simulink model "s20260512_1_quadraped_standup_walk_simulink"  (R2025a)
settings: Solver=FixedStepAuto  StartTime=0.0  StopTime=20  FixedStep=0.001  MaxStep=0.01  RelTol=1e-3
StartFcn:
  | clear functions
values from neighbouring files (symbols this model uses):
  N = size(qr,2)    [animateQuadruped.m]    (also in animateQuadrupedFast.m; animateQuadrupedFastToVideo.m; animateQuadrupedToVideo.m)
  s = norm(axis)    [drawContinuumRobotInstance.m]
  X = 0    [IK_onlyXY.m]    (also in drawContinuumRobotInstance.m = reshape(pts(1,:), size(XC)) + p0(1))
  Y = 0    [IK_onlyXY.m]    (also in drawContinuumRobotInstance.m = reshape(pts(2,:), size(YC)) + p0(2))
  Z = reshape(pts(3,:), size(ZC)) + p0(3)    [drawContinuumRobotInstance.m]
undefined symbols (not defined in the file or in its folder): body_config, leg1_config, leg2_config, leg3_config, leg4_config
libraries: sm_lib x28, nesl_utility x11, simulink x10, snake_single_module_library x5
settings Model: Creator=dperera  LastModifiedBy=dperera
settings SolverCC: ShapePreserveControl=EnableAll  EnableFixedStepZeroCrossing=on
settings OptimizationCC: SimCompilerOptimization=on
settings SFSimCC: UsePrecompiledLibraries=Avoid  SimHardwareAcceleration=native  SimTargetLang=C++  GPUAcceleration=on  SimDLTargetLibrary=cudnn
settings RTWCC: GPUComputeCapability=3.5

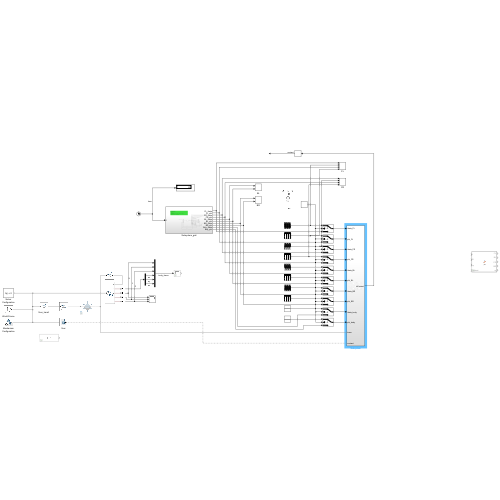
[thumbnail: Simulink's stored preview of the top-level diagram]
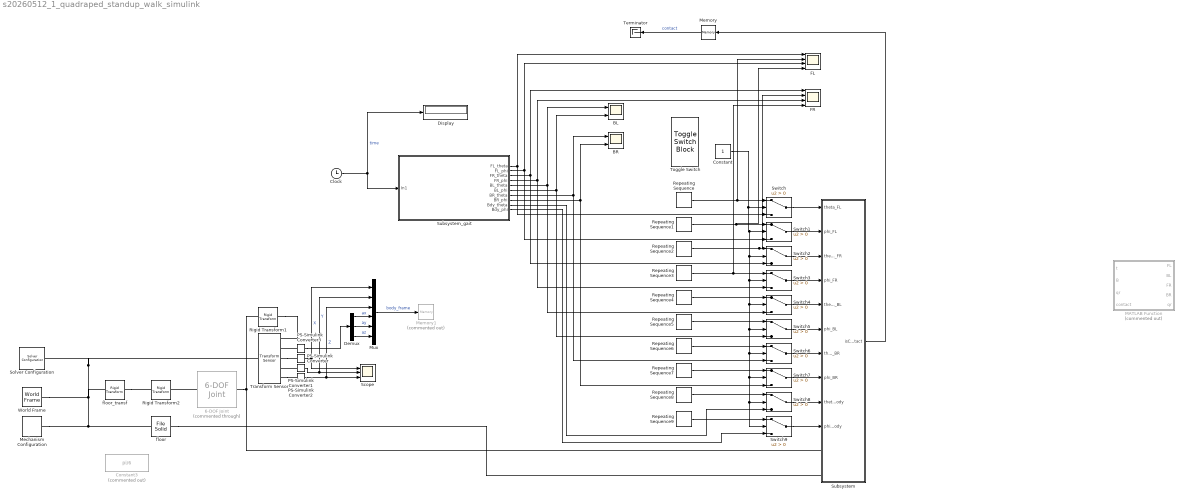
== system s20260512_1_quadraped_standup_walk_simulink ==
  6-DOF Joint : sm_lib/Joints/6-DOF Joint  Commented=through  JointMode=Normal  CompositeWrenchDir=FollowerOnBase  CompositeWrenchFrame=BaseFrame  SenseConstraintForce=off  SenseConstraintTorque=off  SenseTotalForce=off  SenseTotalTorque=off  PxPositionTargetSpecify=off  PxPositionTargetPriority=High  PxPositionTargetValue=0  PxPositionTargetValueUnits=m  PxVelocityTargetSpecify=off  PxVelocityTargetPriority=High  PxVelocityTargetValue=0  PxVelocityTargetValueUnits=m/s  PxEquilibriumPosition=0  PxEquilibriumPositionUnits=m  PxSpringStiffness=0  PxSpringStiffnessUnits=N/m  PxDampingCoefficient=0  PxDampingCoefficientUnits=N/(m/s)  PxLowerLimitSpecify=off  PxLowerLimitBound=-1  PxLowerLimitBoundUnits=m  PxLowerLimitStiffness=1e6  PxLowerLimitStiffnessUnits=N/m  PxLowerLimitDamping=1e3  PxLowerLimitDampingUnits=N/(m/s)  PxLowerLimitTransitionRegionWidth=1e-4  PxLowerLimitTransitionRegionWidthUnits=m  PxUpperLimitSpecify=off  PxUpperLimitBound=1  PxUpperLimitBoundUnits=m  PxUpperLimitStiffness=1e6  PxUpperLimitStiffnessUnits=N/m  PxUpperLimitDamping=1e3  PxUpperLimitDampingUnits=N/(m/s)  PxUpperLimitTransitionRegionWidth=1e-4  PxUpperLimitTransitionRegionWidthUnits=m  PxTorqueActuationMode=NoTorque  PxMotionActuationMode=ComputedMotion  PxSensePosition=off  PxSenseVelocity=off  PxSenseAcceleration=off  PxSenseTorqueForce=off  PxSenseLowerLimitTorqueForce=off  PxSenseUpperLimitTorqueForce=off  PyPositionTargetSpecify=off  PyPositionTargetPriority=High  PyPositionTargetValue=0  PyPositionTargetValueUnits=m  PyVelocityTargetSpecify=off  PyVelocityTargetPriority=High  PyVelocityTargetValue=0  PyVelocityTargetValueUnits=m/s  PyEquilibriumPosition=0  PyEquilibriumPositionUnits=m  PySpringStiffness=0  PySpringStiffnessUnits=N/m  PyDampingCoefficient=0  PyDampingCoefficientUnits=N/(m/s)  PyLowerLimitSpecify=off  PyLowerLimitBound=-1  PyLowerLimitBoundUnits=m  PyLowerLimitStiffness=1e6  PyLowerLimitStiffnessUnits=N/m  PyLowerLimitDamping=1e3  PyLowerLimitDampingUnits=N/(m/s)  PyLowerLimitTransitionRegionWidth=1e-4  PyLowerLimitTransitionRegionWidthUnits=m  PyUpperLimitSpecify=off  PyUpperLimitBound=1  PyUpperLimitBoundUnits=m  PyUpperLimitStiffness=1e6  PyUpperLimitStiffnessUnits=N/m  PyUpperLimitDamping=1e3  PyUpperLimitDampingUnits=N/(m/s)  PyUpperLimitTransitionRegionWidth=1e-4  PyUpperLimitTransitionRegionWidthUnits=m  PyTorqueActuationMode=NoTorque  PyMotionActuationMode=ComputedMotion  PySensePosition=off  PySenseVelocity=off  PySenseAcceleration=off  PySenseTorqueForce=off  PySenseLowerLimitTorqueForce=off  PySenseUpperLimitTorqueForce=off  PzPositionTargetSpecify=off  PzPositionTargetPriority=High  PzPositionTargetValue=0  PzPositionTargetValueUnits=m  PzVelocityTargetSpecify=off  PzVelocityTargetPriority=High  PzVelocityTargetValue=0  PzVelocityTargetValueUnits=m/s  PzEquilibriumPosition=0  PzEquilibriumPositionUnits=m  PzSpringStiffness=0  PzSpringStiffnessUnits=N/m  PzDampingCoefficient=0  PzDampingCoefficientUnits=N/(m/s)  PzLowerLimitSpecify=off  PzLowerLimitBound=-1  PzLowerLimitBoundUnits=m  PzLowerLimitStiffness=1e6  PzLowerLimitStiffnessUnits=N/m  PzLowerLimitDamping=1e3  PzLowerLimitDampingUnits=N/(m/s)  PzLowerLimitTransitionRegionWidth=1e-4  PzLowerLimitTransitionRegionWidthUnits=m  PzUpperLimitSpecify=off  PzUpperLimitBound=1  PzUpperLimitBoundUnits=m  PzUpperLimitStiffness=1e6  PzUpperLimitStiffnessUnits=N/m  PzUpperLimitDamping=1e3  PzUpperLimitDampingUnits=N/(m/s)  PzUpperLimitTransitionRegionWidth=1e-4  PzUpperLimitTransitionRegionWidthUnits=m  PzTorqueActuationMode=NoTorque  PzMotionActuationMode=ComputedMotion  PzSensePosition=off  PzSenseVelocity=off  PzSenseAcceleration=off  PzSenseTorqueForce=off  PzSenseLowerLimitTorqueForce=off  PzSenseUpperLimitTorqueForce=off  SphPositionTargetSpecify=off  SphPositionTargetPriority=High  SphPositionTargetRotationMethod=None  SphPositionTargetFollAlignAxisA=+X  SphPositionTargetBaseAlignAxisA=+Y  SphPositionTargetFollAlignAxisB=+Y  SphPositionTargetBaseAlignAxisB=+Z  SphPositionTargetRotationStandardAxis=+Z  SphPositionTargetRotationAngle=0  SphPositionTargetRotationAngleUnits=deg  SphPositionTargetRotationArbitraryAxis=[0 0 1]  SphPositionTargetRotationSequenceAxes=FollowerAxes  SphPositionTargetRotationSequence=XYX  SphPositionTargetRotationSequenceAngles=[0 0 0]  SphPositionTargetRotationSequenceAnglesUnits=deg  SphPositionTargetRotationMatrix=[1 0 0;0 1 0;0 0 1]  SphPositionTargetQuaternion=[1 0 0 0]  SphVelocityTargetSpecify=off  SphVelocityTargetPriority=High  SphVelocityTargetValue=[0 0 0]  SphVelocityTargetValueUnits=deg/s  SphVelocityTargetInFollowerFrame=on  SphEqPosRotationMethod=None  SphEqPosFollAlignAxisA=+X  SphEqPosBaseAlignAxisA=+Y  SphEqPosFollAlignAxisB=+Y  SphEqPosBaseAlignAxisB=+Z  SphEqPosRotationStandardAxis=+Z  SphEqPosRotationAngle=0  SphEqPosRotationAngleUnits=deg  SphEqPosRotationArbitraryAxis=[0 0 1]  SphEqPosRotationSequenceAxes=FollowerAxes  SphEqPosRotationSequence=XYX  SphEqPosRotationSequenceAngles=[0 0 0]  SphEqPosRotationSequenceAnglesUnits=deg  SphEqPosRotationMatrix=[1 0 0;0 1 0;0 0 1]  SphEqPosQuaternion=[1 0 0 0]  SphSpringStiffness=0  SphSpringStiffnessUnits=N*m/deg  SphDampingCoefficient=0  SphDampingCoefficientUnits=N*m/(deg/s)  SphLowerLimitSpecify=off  SphLowerLimitBound=15  SphLowerLimitBoundUnits=deg  SphLowerLimitStiffness=1e4  SphLowerLimitStiffnessUnits=N*m/deg  SphLowerLimitDamping=10  SphLowerLimitDampingUnits=N*m/(deg/s)  SphLowerLimitTransitionRegionWidth=0.1  SphLowerLimitTransitionRegionWidthUnits=deg  SphUpperLimitSpecify=off  SphUpperLimitBound=45  SphUpperLimitBoundUnits=deg  SphUpperLimitStiffness=1e4  SphUpperLimitStiffnessUnits=N*m/deg  SphUpperLimitDamping=10  SphUpperLimitDampingUnits=N*m/(deg/s)  SphUpperLimitTransitionRegionWidth=0.1  SphUpperLimitTransitionRegionWidthUnits=deg  SphTorqueActuationMode=NoTorque  SphActuateTorqueX=off  SphActuateTorqueY=off  SphActuateTorqueZ=off  SphActuateTorque=off  SphActuationFrame=BaseFrame  SphSensePosition=off  SphSenseVelocityX=off  SphSenseVelocityY=off  SphSenseVelocityZ=off  SphSenseVelocity=off  SphSenseAccelerationX=off  SphSenseAccelerationY=off  SphSenseAccelerationZ=off  SphSenseAcceleration=off  SphSenseLowerLimitTorqueMag=off  SphSenseUpperLimitTorqueMag=off  SphSensingFrame=BaseFrame
  BL : Scope  NumInputPorts=2
      settings: ActiveDisplayYMinimum=-0.20716237469260496  ActiveDisplayYMaximum=1.6983723206609396  DataLoggingVariableName=ScopeData2
  BR : Scope  NumInputPorts=2
      settings: ActiveDisplayYMinimum=-0.17908356441991335  ActiveDisplayYMaximum=1.6117480671745472  DataLoggingVariableName=ScopeData4
  Clock : Clock
  Constant : Constant
  Constant3 : Constant  Commented=on  Value=pi/6
  Demux : Demux  Outputs=3
  Display : Display
  FL : Scope  NumInputPorts=4
      settings: ActiveDisplayYMinimum=-0.21837167483905506  ActiveDisplayYMaximum=1.9654509962748026
  FR : Scope  NumInputPorts=4
      settings: ActiveDisplayYMinimum=-0.31265338262436854  ActiveDisplayYMaximum=1.8657324459490972  DataLoggingVariableName=ScopeData3
  MATLAB Function : MATLAB Function  Commented=on  TreatAsAtomicUnit=on
  Mechanism Configuration : sm_lib/Utilities/Mechanism Configuration  UniformGravity=Constant  GravityVector=[0 0 -9.8067]  GravityVectorUnits=m/s^2  LinearizationDelta=0.001  JointModeTransitionNonlinearIterations=2
  Memory : Memory
  Memory1 : Memory  Commented=on  InitialCondition=[0;0;0.25;0;0;0]
  Mux : Mux  Inputs=6
  PS-Simulink Converter{,1..3} (4 alike) : nesl_utility/PS-Simulink Converter  PhysicalDomain=network_engine_domain  SubClassName=ps_output  LeftPortType=input  RightPortType=output  PseudoPeriodic=off  Frequencies=[]  VectorFormat=inherit  Unit=inherit  AffineConversion=off
  Repeating Sequence : simulink/Sources/Repeating Sequence  rep_seq_t=t  rep_seq_y=leg1_config(1,:)
  Repeating Sequence1 : simulink/Sources/Repeating Sequence  rep_seq_t=t  rep_seq_y=leg1_config(2,:)
  Repeating Sequence2 : simulink/Sources/Repeating Sequence  rep_seq_t=t  rep_seq_y=leg3_config(1,:)
  Repeating Sequence3 : simulink/Sources/Repeating Sequence  rep_seq_t=t  rep_seq_y=leg3_config(2,:)
  Repeating Sequence4 : simulink/Sources/Repeating Sequence  rep_seq_t=t  rep_seq_y=leg2_config(1,:)
  Repeating Sequence5 : simulink/Sources/Repeating Sequence  rep_seq_t=t  rep_seq_y=leg2_config(2,:)
  Repeating Sequence6 : simulink/Sources/Repeating Sequence  rep_seq_t=t  rep_seq_y=leg4_config(1,:)
  Repeating Sequence7 : simulink/Sources/Repeating Sequence  rep_seq_t=t  rep_seq_y=leg4_config(2,:)
  Repeating Sequence8 : simulink/Sources/Repeating Sequence  rep_seq_t=t  rep_seq_y=body_config(1,:)
  Repeating Sequence9 : simulink/Sources/Repeating Sequence  rep_seq_t=t  rep_seq_y=body_config(2,:)
  Rigid Transform1 : sm_lib/Frames and Transforms/Rigid Transform  RotationMethod=StandardAxis  FollAlignAxisA=+X  BaseAlignAxisA=+Y  FollAlignAxisB=+Y  BaseAlignAxisB=+Z  RotationStandardAxis=+Z  RotationAngle=-pi/2  RotationAngleUnits=rad  RotationArbitraryAxis=[0 0 1]  RotationSequenceAxes=FollowerAxes  RotationSequence=XYX  RotationSequenceAngles=[0 0 0]  RotationSequenceAnglesUnits=deg  RotationMatrix=[1 0 0;0 1 0;0 0 1]  Quaternion=[1 0 0 0]  TranslationMethod=None  TranslationCartesianOffset=[-1.5 -.40 0.790/2+0.025]  TranslationCartesianOffsetUnits=m  TranslationStandardAxis=+Z  TranslationStandardOffset=0.035  TranslationStandardOffsetUnits=m  TranslationROffset=0  TranslationROffsetUnits=m  TranslationThetaOffset=0  TranslationThetaOffsetUnits=deg  TranslationZOffset=0  TranslationZOffsetUnits=m
  Rigid Transform2 : sm_lib/Frames and Transforms/Rigid Transform  RotationMethod=StandardAxis  FollAlignAxisA=+X  BaseAlignAxisA=+Y  FollAlignAxisB=+Y  BaseAlignAxisB=+Z  RotationStandardAxis=+Z  RotationAngle=pi/2  RotationAngleUnits=rad  RotationArbitraryAxis=[0 0 1]  RotationSequenceAxes=FollowerAxes  RotationSequence=XYX  RotationSequenceAngles=[0 0 0]  RotationSequenceAnglesUnits=deg  RotationMatrix=[1 0 0;0 1 0;0 0 1]  Quaternion=[1 0 0 0]  TranslationMethod=None  TranslationCartesianOffset=[-1.5 -.40 0.790/2+0.025]  TranslationCartesianOffsetUnits=m  TranslationStandardAxis=+Z  TranslationStandardOffset=0.035  TranslationStandardOffsetUnits=m  TranslationROffset=0  TranslationROffsetUnits=m  TranslationThetaOffset=0  TranslationThetaOffsetUnits=deg  TranslationZOffset=0  TranslationZOffsetUnits=m
  Scope : Scope  NumInputPorts=3
      settings: ActiveDisplayYMinimum=-0.054501031030468931  ActiveDisplayYMaximum=0.41653003082846396
  Solver Configuration : nesl_utility/Solver Configuration  PhysicalDomain=network_engine_domain  SubClassName=solver  LeftPortType=input  RightPortType=generic  Tones=[]  Harmonics=[]  SimulateNoise=off  Profile=off  UseLocalSampling=off  EnableSwitchedLinearOptims=on  FrequencyDomain=off  UseCCode=off  RelTol=0.001  AbsTol=1e-06  MinStep=1e-09  ToWorkspace=off  RevertToSquareIcSolve=off  NumHomotopyIterations=100  PhasorMode=off  PhasorModeNumHarmonics=1  ConsistencySolver=NEWTON_XTOL_AFTER_FTOL  IndexReductionMethod=DerivativeReplacement  DoDC=off  ResidualTolerance=1e-09  ConsistencyTolSource=GLOBAL  ConsistencyAbsTol=0.001  ConsistencyRelTol=0.001  ConsistencyTolFactor=0.001  UseLocalSolver=off  LocalSolverChoice=NE_BACKWARD_EULER_ADVANCER  ResolveIndetEquations=on  FunctionEvalNumThread=1  LocalSolverSampleTime=0.001  DoFixedCost=off  MaxNonlinIter=3  MaxModeIter=2  ComputeImpulses=off  ImpulseIterations=2  LinearAlgebra=Sparse  LinearAlgebraNumThread=0  EquationFormulation=NE_TIME_EF  DelaysMemoryBudget=1024  AutomaticFiltering=on  FilteringTimeConstant=0.001  PartitionStorageMethod=AS_NEEDED  PartitionMemoryBudget=1024  PartitionMethod=FAST  MultibodyUseLocalSolver=off  MultibodyLocalSolverChoice=ODE8  MultibodyLocalSolverSampleTime=0.001
  Subsystem : Subsystem
  Subsystem_gait : Subsystem
  Switch{,1..9} (10 alike) : Switch  Criteria=u2 > Threshold  SaturateOnIntegerOverflow=off  InputSameDT=off
  Terminator : Terminator
  Toggle Switch : ToggleSwitchBlock
  Transform Sensor : sm_lib/Frames and Transforms/Transform Sensor  MeasurementFrame=World  RotationSequence=XYZ  SenseAngle=off  SenseAxis=off  SenseQ=off  SenseR=off  SenseRotationSequence=on  SenseOmegaX=off  SenseOmegaY=off  SenseOmegaZ=off  SenseOmega=off  SenseQDot=off  SenseRDot=off  SenseRotationSequenceDot=off  SenseAlphaX=off  SenseAlphaY=off  SenseAlphaZ=off  SenseAlpha=off  SenseQDDot=off  SenseRDDot=off  SenseX=on  SenseY=on  SenseZ=on  SenseXYZ=off  SenseRad=off  SenseAzim=off  SenseDist=off  SenseInc=off  SenseXDot=off  SenseYDot=off  SenseZDot=off  SenseXYZDot=off  SenseRadDot=off  SenseAzimDot=off  SenseDistDot=off  SenseIncDot=off  SenseXDDot=off  SenseYDDot=off  SenseZDDot=off  SenseXYZDDot=off  SenseRadDDot=off  SenseAzimDDot=off  SenseDistDDot=off  SenseIncDDot=off
  World Frame : sm_lib/Frames and Transforms/World Frame
  floor : sm_lib/Body Elements/File Solid  ExtGeomFileName=C:\Users\dperera\OneDrive - Texas A&M University\Byrd, Nathan Chandler's files - Snake Locomotion\Snake_Locomotion_Matlab\Snake_Locomotion_Solidworks\floor.STEP  UnitType=FromFile  ExtGeomFileUnits=m  StepReaderType=HEX  ExportConvexHullGeometry=on  InertiaType=CalculateFromGeometry  BasedOnType=Density  Density=1000000  DensityUnits=kg/m^3  Mass=10  MassUnits=g  CenterOfMass=[0 0 0]  CenterOfMassUnits=m  MomentsOfInertia=[1 1 1]  MomentsOfInertiaUnits=kg*m^2  ProductsOfInertia=[0 0 0]  ProductsOfInertiaUnits=kg*m^2  GraphicType=FromGeometry  MarkerShape=Sphere  MarkerSize=10  GraphicVisPropType=AdvancedVisualProperties  GraphicDiffuseColor=[0.6275 0.6275 0.6275]  GraphicOpacity=1  GraphicSpecularColor=[0.5 0.5 0.5 1.0]  GraphicAmbientColor=[0.15 0.15 0.15 1.0]  GraphicEmissiveColor=[0.0 0.0 0.0 1.0]  GraphicShininess=10  DoExposeReferenceFrame=off  SerializedFrames=<Frames><Frame><Id>Frame1</Id><Value><Name>F1</Name><Origin><Source>ReferenceFrame</Source><FeatureName></FeatureName></Origin><PrimaryAxis><DefinedDirection>+Z</DefinedDirection><Source>ReferenceFrame</Source><SourceDirection>+Z</SourceDirection><FeatureName></FeatureName></PrimaryAxis><SecondaryAxis><DefinedDirection>+X</DefinedDirection><Source>ReferenceFrame</Source><SourceDirection>+X</SourceDirection><FeatureName></FeatureName></SecondaryAxis></Value></Frame></Frames>
  floor_transf : sm_lib/Frames and Transforms/Rigid Transform  RotationMethod=None  FollAlignAxisA=+X  BaseAlignAxisA=+Y  FollAlignAxisB=+Y  BaseAlignAxisB=+Z  RotationStandardAxis=+Z  RotationAngle=0  RotationAngleUnits=deg  RotationArbitraryAxis=[0 0 1]  RotationSequenceAxes=FollowerAxes  RotationSequence=XYX  RotationSequenceAngles=[0 0 0]  RotationSequenceAnglesUnits=deg  RotationMatrix=[1 0 0;0 1 0;0 0 1]  Quaternion=[1 0 0 0]  TranslationMethod=Cartesian  TranslationCartesianOffset=[0.0, 0.0, 0.535]  TranslationCartesianOffsetUnits=m  TranslationStandardAxis=+Z  TranslationStandardOffset=0.0326  TranslationStandardOffsetUnits=m  TranslationROffset=0  TranslationROffsetUnits=m  TranslationThetaOffset=0  TranslationThetaOffsetUnits=deg  TranslationZOffset=0  TranslationZOffsetUnits=m
  wires:
  PS-Simulink Converter/1 -> Scope/1, Mux/1  "X"
  PS-Simulink Converter1/1 -> Scope/2, Mux/2  "Y"
  PS-Simulink Converter2/1 -> Mux/3, Scope/3  "Z"
  PS-Simulink Converter3/1 -> Demux/1
  Demux/1 -> Mux/4  "ax"
  Demux/2 -> Mux/5  "ay"
  Demux/3 -> Mux/6  "az"
  Clock/1 -> Display/1, Subsystem_gait/1(In1)  "time"
  Mux/1 -> Memory1/1  "body_frame"
  Subsystem/1(isContact) -> Memory/1
  Subsystem_gait/1(FL_theta) -> Switch/3, FL/1
  Subsystem_gait/2(FL_phi) -> Switch1/3, FL/3
  Subsystem_gait/3(FR_theta) -> Switch2/3, FR/1
  Subsystem_gait/4(FR_phi) -> Switch3/3, FR/3
  Subsystem_gait/5(BL_theta) -> BL/1, Switch4/3
  Subsystem_gait/6(BL_phi) -> Switch5/3, BL/2
  Subsystem_gait/7(BR_theta) -> Switch6/3, BR/1
  Subsystem_gait/8(BR_phi) -> Switch7/3, BR/2
  Switch/1 -> Subsystem/1(theta_FL)
  Switch1/1 -> Subsystem/2(phi_FL)
  Switch2/1 -> Subsystem/3(theta_FR)
  Switch3/1 -> Subsystem/4(phi_FR)
  Switch4/1 -> Subsystem/5(theta_BL)
  Switch5/1 -> Subsystem/6(phi_BL)
  Switch6/1 -> Subsystem/7(theta_BR)
  Switch7/1 -> Subsystem/8(phi_BR)
  Switch8/1 -> Subsystem/9(theta_body)
  Switch9/1 -> Subsystem/10(phi_body)
  Subsystem_gait/10(Bdy_phi) -> Switch9/3
  Subsystem_gait/9(Bdy_theta) -> Switch8/3
  Repeating Sequence/1 -> FL/2, Switch/1
  Repeating Sequence1/1 -> FL/4, Switch1/1
  Repeating Sequence2/1 -> FR/2, Switch2/1
  Repeating Sequence3/1 -> FR/4, Switch3/1
  Repeating Sequence4/1 -> Switch4/1
  Repeating Sequence5/1 -> Switch5/1
  Repeating Sequence6/1 -> Switch6/1
  Repeating Sequence9/1 -> Switch9/1
  Repeating Sequence8/1 -> Switch8/1
  Repeating Sequence7/1 -> Switch7/1
  Constant/1 -> Switch9/2, Switch8/2, Switch7/2, Switch6/2, Switch5/2, Switch4/2, Switch3/2, Switch2/2, Switch1/2, Switch/2
  Memory/1 -> Terminator/1  "contact"
  connections:
  floor_transf/RConn1 -- Rigid Transform2/LConn1
  Mechanism Configuration/RConn1 -- Transform Sensor/LConn1 -- Solver Configuration/RConn1 -- floor_transf/LConn1 -- World Frame/RConn1 -- floor/LConn1
  6-DOF Joint/LConn1 -- Rigid Transform2/RConn1
  6-DOF Joint/RConn1 -- Subsystem/LConn1 -- Rigid Transform1/LConn1
  floor/RConn1 -- Subsystem/LConn2
  Transform Sensor/RConn3 -- PS-Simulink Converter/LConn1
  PS-Simulink Converter1/LConn1 -- Transform Sensor/RConn4
  Transform Sensor/RConn5 -- PS-Simulink Converter2/LConn1
  PS-Simulink Converter3/LConn1 -- Transform Sensor/RConn2
  Rigid Transform1/RConn1 -- Transform Sensor/RConn1

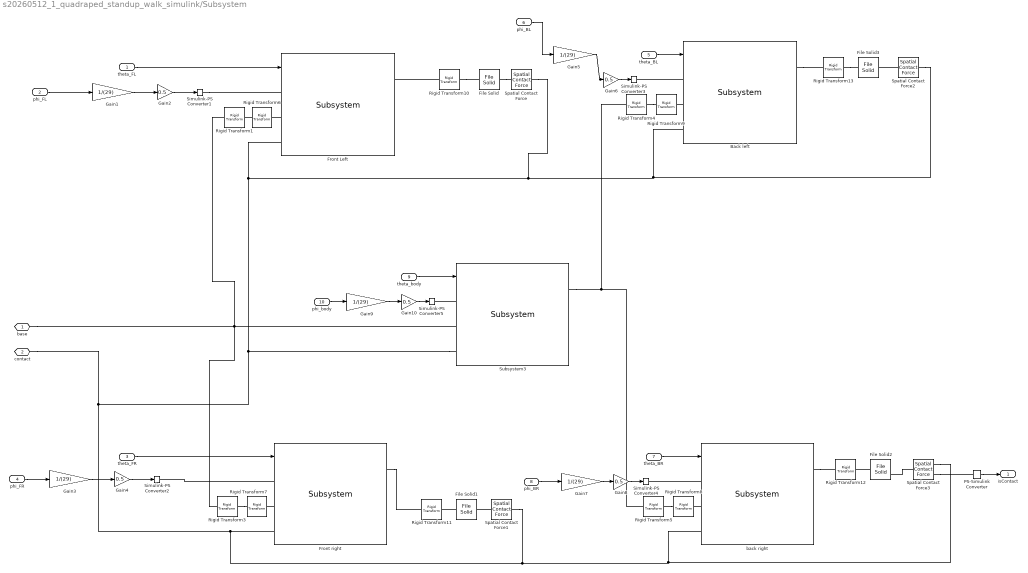
== system s20260512_1_quadraped_standup_walk_simulink/Subsystem ==
  theta_FL : Inport
  phi_FL : Inport  Port=2
  theta_FR : Inport  Port=3
  phi_FR : Inport  Port=4
  theta_BL : Inport  Port=5
  phi_BL : Inport  Port=6
  theta_BR : Inport  Port=7
  phi_BR : Inport  Port=8
  theta_body : Inport  Port=9
  phi_body : Inport  Port=10
  Back left : snake_single_module_library/Subsystem  SystemSampleTime=-1  VariantActivationTime=update diagram  EmptyChoice=off  PassThrough=off  PassThroughVariantControl=(default)  EmptyChoiceVariantControl=(default)  AllowFlexibleInterface=on  Latency=0  AutoFrameSizeCalculation=off
  File Solid : sm_lib/Body Elements/File Solid  ExtGeomFileName=\solidworks\foot_tip.STEP  UnitType=FromFile  ExtGeomFileUnits=m  StepReaderType=HEX  ExportConvexHullGeometry=on  InertiaType=CalculateFromGeometry  BasedOnType=Mass  Density=1000  DensityUnits=kg/m^3  Mass=0.1  MassUnits=kg  CenterOfMass=[0 0 0]  CenterOfMassUnits=m  MomentsOfInertia=[1 1 1]  MomentsOfInertiaUnits=kg*m^2  ProductsOfInertia=[0 0 0]  ProductsOfInertiaUnits=kg*m^2  GraphicType=FromGeometry  MarkerShape=Sphere  MarkerSize=10  GraphicVisPropType=SimpleVisualProperties  GraphicDiffuseColor=[0.3333 0.6667 0]  GraphicOpacity=1  GraphicSpecularColor=[0.5 0.5 0.5 1.0]  GraphicAmbientColor=[0.15 0.15 0.15 1.0]  GraphicEmissiveColor=[0.0 0.0 0.0 1.0]  GraphicShininess=75  DoExposeReferenceFrame=off  SerializedFrames=<Frames><Frame><Id>Frame1</Id><Value><Name>F1</Name><Origin><Source>ReferenceFrame</Source><FeatureName></FeatureName></Origin><PrimaryAxis><DefinedDirection>+Z</DefinedDirection><Source>ReferenceFrame</Source><SourceDirection>+Z</SourceDirection><FeatureName></FeatureName></PrimaryAxis><SecondaryAxis><DefinedDirection>+X</DefinedDirection><Source>ReferenceFrame</Source><SourceDirection>+X</SourceDirection><FeatureName></FeatureName></SecondaryAxis></Value></Frame></Frames>
  File Solid1 : sm_lib/Body Elements/File Solid  ExtGeomFileName=\solidworks\foot_tip.STEP  UnitType=FromFile  ExtGeomFileUnits=m  StepReaderType=HEX  ExportConvexHullGeometry=on  InertiaType=CalculateFromGeometry  BasedOnType=Mass  Density=1000  DensityUnits=kg/m^3  Mass=0.1  MassUnits=kg  CenterOfMass=[0 0 0]  CenterOfMassUnits=m  MomentsOfInertia=[1 1 1]  MomentsOfInertiaUnits=kg*m^2  ProductsOfInertia=[0 0 0]  ProductsOfInertiaUnits=kg*m^2  GraphicType=FromGeometry  MarkerShape=Sphere  MarkerSize=10  GraphicVisPropType=SimpleVisualProperties  GraphicDiffuseColor=[0.3333 0.6667 0]  GraphicOpacity=1  GraphicSpecularColor=[0.5 0.5 0.5 1.0]  GraphicAmbientColor=[0.15 0.15 0.15 1.0]  GraphicEmissiveColor=[0.0 0.0 0.0 1.0]  GraphicShininess=75  DoExposeReferenceFrame=on  SerializedFrames=<Frames/>
  File Solid2 : sm_lib/Body Elements/File Solid  ExtGeomFileName=\solidworks\foot_tip.STEP  UnitType=FromFile  ExtGeomFileUnits=m  StepReaderType=HEX  ExportConvexHullGeometry=on  InertiaType=CalculateFromGeometry  BasedOnType=Mass  Density=1000  DensityUnits=kg/m^3  Mass=0.1  MassUnits=kg  CenterOfMass=[0 0 0]  CenterOfMassUnits=m  MomentsOfInertia=[1 1 1]  MomentsOfInertiaUnits=kg*m^2  ProductsOfInertia=[0 0 0]  ProductsOfInertiaUnits=kg*m^2  GraphicType=FromGeometry  MarkerShape=Sphere  MarkerSize=10  GraphicVisPropType=SimpleVisualProperties  GraphicDiffuseColor=[0.3333 0.6667 0]  GraphicOpacity=1  GraphicSpecularColor=[0.5 0.5 0.5 1.0]  GraphicAmbientColor=[0.15 0.15 0.15 1.0]  GraphicEmissiveColor=[0.0 0.0 0.0 1.0]  GraphicShininess=75  DoExposeReferenceFrame=on  SerializedFrames=<Frames><Frame><Id>Frame1</Id><Value><Name>tip</Name><Origin><Source>GeometricFeature</Source><FeatureName>point 2</FeatureName></Origin><PrimaryAxis><DefinedDirection>+Z</DefinedDirection><Source>ReferenceFrame</Source><SourceDirection>+Z</SourceDirection><FeatureName></FeatureName></PrimaryAxis><SecondaryAxis><DefinedDirection>+X</DefinedDirection><Source>ReferenceFrame</Source><SourceDirection>+X</SourceDirection><FeatureName></FeatureName></SecondaryAxis></Value></Frame></Frames>
  File Solid3 : sm_lib/Body Elements/File Solid  ExtGeomFileName=\solidworks\foot_tip.STEP  UnitType=FromFile  ExtGeomFileUnits=m  StepReaderType=HEX  ExportConvexHullGeometry=on  InertiaType=CalculateFromGeometry  BasedOnType=Mass  Density=1000  DensityUnits=kg/m^3  Mass=0.1  MassUnits=kg  CenterOfMass=[0 0 0]  CenterOfMassUnits=m  MomentsOfInertia=[1 1 1]  MomentsOfInertiaUnits=kg*m^2  ProductsOfInertia=[0 0 0]  ProductsOfInertiaUnits=kg*m^2  GraphicType=FromGeometry  MarkerShape=Sphere  MarkerSize=10  GraphicVisPropType=SimpleVisualProperties  GraphicDiffuseColor=[0.3333 0.6667 0]  GraphicOpacity=1  GraphicSpecularColor=[0.5 0.5 0.5 1.0]  GraphicAmbientColor=[0.15 0.15 0.15 1.0]  GraphicEmissiveColor=[0.0 0.0 0.0 1.0]  GraphicShininess=75  DoExposeReferenceFrame=on  SerializedFrames=<Frames/>
  Front Left : snake_single_module_library/Subsystem  SystemSampleTime=-1  VariantActivationTime=update diagram  EmptyChoice=off  PassThrough=off  PassThroughVariantControl=(default)  EmptyChoiceVariantControl=(default)  AllowFlexibleInterface=on  Latency=0  AutoFrameSizeCalculation=off
  Front right : snake_single_module_library/Subsystem  SystemSampleTime=-1  VariantActivationTime=update diagram  EmptyChoice=off  PassThrough=off  PassThroughVariantControl=(default)  EmptyChoiceVariantControl=(default)  AllowFlexibleInterface=on  Latency=0  AutoFrameSizeCalculation=off
  Gain{1,3,5,7,9} (5 alike) : Gain  Gain=1/(29)
  Gain{2,4,6,8,10} (5 alike) : Gain  Gain=0.5
  PS-Simulink Converter : nesl_utility/PS-Simulink Converter  PhysicalDomain=network_engine_domain  SubClassName=ps_output  LeftPortType=input  RightPortType=output  PseudoPeriodic=off  Frequencies=[]  VectorFormat=inherit  Unit=inherit  AffineConversion=off
  Rigid Transform1 : sm_lib/Frames and Transforms/Rigid Transform  RotationMethod=StandardAxis  FollAlignAxisA=+X  BaseAlignAxisA=+Y  FollAlignAxisB=+Y  BaseAlignAxisB=+Z  RotationStandardAxis=+Z  RotationAngle=-pi/2  RotationAngleUnits=rad  RotationArbitraryAxis=[0 0 1]  RotationSequenceAxes=FollowerAxes  RotationSequence=XYX  RotationSequenceAngles=[0 0 0]  RotationSequenceAnglesUnits=rad  RotationMatrix=[1 0 0;0 1 0;0 0 1]  Quaternion=[1 0 0 0]  TranslationMethod=Cartesian  TranslationCartesianOffset=[0.03; -0.025; 0.0]  TranslationCartesianOffsetUnits=m  TranslationStandardAxis=+X  TranslationStandardOffset=0.035  TranslationStandardOffsetUnits=m  TranslationROffset=0  TranslationROffsetUnits=m  TranslationThetaOffset=0  TranslationThetaOffsetUnits=deg  TranslationZOffset=0  TranslationZOffsetUnits=m
  Rigid Transform{10..13} (4 alike) : sm_lib/Frames and Transforms/Rigid Transform  RotationMethod=StandardAxis  FollAlignAxisA=+X  BaseAlignAxisA=+Y  FollAlignAxisB=+Y  BaseAlignAxisB=+Z  RotationStandardAxis=+X  RotationAngle=-pi/2  RotationAngleUnits=rad  RotationArbitraryAxis=[0 0 1]  RotationSequenceAxes=FollowerAxes  RotationSequence=XYX  RotationSequenceAngles=[0 0 0]  RotationSequenceAnglesUnits=rad  RotationMatrix=[1 0 0;0 1 0;0 0 1]  Quaternion=[1 0 0 0]  TranslationMethod=None  TranslationCartesianOffset=[0.03; -0.025; 0.0]  TranslationCartesianOffsetUnits=m  TranslationStandardAxis=+X  TranslationStandardOffset=0.035  TranslationStandardOffsetUnits=m  TranslationROffset=0  TranslationROffsetUnits=m  TranslationThetaOffset=0  TranslationThetaOffsetUnits=deg  TranslationZOffset=0  TranslationZOffsetUnits=m
  Rigid Transform3 : sm_lib/Frames and Transforms/Rigid Transform  RotationMethod=StandardAxis  FollAlignAxisA=+X  BaseAlignAxisA=+Y  FollAlignAxisB=+Y  BaseAlignAxisB=+Z  RotationStandardAxis=+Z  RotationAngle=pi/2  RotationAngleUnits=rad  RotationArbitraryAxis=[0 0 1]  RotationSequenceAxes=FollowerAxes  RotationSequence=XYX  RotationSequenceAngles=[0 0 0]  RotationSequenceAnglesUnits=deg  RotationMatrix=[1 0 0;0 1 0;0 0 1]  Quaternion=[1 0 0 0]  TranslationMethod=Cartesian  TranslationCartesianOffset=[-0.03; -0.025; 0.0]  TranslationCartesianOffsetUnits=m  TranslationStandardAxis=+X  TranslationStandardOffset=0.035  TranslationStandardOffsetUnits=m  TranslationROffset=0  TranslationROffsetUnits=m  TranslationThetaOffset=0  TranslationThetaOffsetUnits=deg  TranslationZOffset=0  TranslationZOffsetUnits=m
  Rigid Transform4 : sm_lib/Frames and Transforms/Rigid Transform  RotationMethod=StandardAxis  FollAlignAxisA=+X  BaseAlignAxisA=+Y  FollAlignAxisB=+Y  BaseAlignAxisB=+Z  RotationStandardAxis=+Z  RotationAngle=-pi/2  RotationAngleUnits=rad  RotationArbitraryAxis=[0 0 1]  RotationSequenceAxes=FollowerAxes  RotationSequence=XYX  RotationSequenceAngles=[0 0 0]  RotationSequenceAnglesUnits=deg  RotationMatrix=[1 0 0;0 1 0;0 0 1]  Quaternion=[1 0 0 0]  TranslationMethod=Cartesian  TranslationCartesianOffset=[0.025; 0.02; 0.0]  TranslationCartesianOffsetUnits=m  TranslationStandardAxis=+X  TranslationStandardOffset=0.035  TranslationStandardOffsetUnits=m  TranslationROffset=0  TranslationROffsetUnits=m  TranslationThetaOffset=0  TranslationThetaOffsetUnits=deg  TranslationZOffset=0  TranslationZOffsetUnits=m
  Rigid Transform5 : sm_lib/Frames and Transforms/Rigid Transform  RotationMethod=StandardAxis  FollAlignAxisA=+X  BaseAlignAxisA=+Y  FollAlignAxisB=+Y  BaseAlignAxisB=+Z  RotationStandardAxis=+Z  RotationAngle=pi/2  RotationAngleUnits=rad  RotationArbitraryAxis=[0 0 1]  RotationSequenceAxes=FollowerAxes  RotationSequence=XYX  RotationSequenceAngles=[0 0 0]  RotationSequenceAnglesUnits=deg  RotationMatrix=[1 0 0;0 1 0;0 0 1]  Quaternion=[1 0 0 0]  TranslationMethod=Cartesian  TranslationCartesianOffset="[-0.025;  0.02; 0.0]"  TranslationCartesianOffsetUnits=m  TranslationStandardAxis=+X  TranslationStandardOffset=0.035  TranslationStandardOffsetUnits=m  TranslationROffset=0  TranslationROffsetUnits=m  TranslationThetaOffset=0  TranslationThetaOffsetUnits=deg  TranslationZOffset=0  TranslationZOffsetUnits=m
  Rigid Transform{6..9} (4 alike) : sm_lib/Frames and Transforms/Rigid Transform  RotationMethod=StandardAxis  FollAlignAxisA=+X  BaseAlignAxisA=+Y  FollAlignAxisB=+Y  BaseAlignAxisB=+Z  RotationStandardAxis=+Y  RotationAngle=-pi/2  RotationAngleUnits=rad  RotationArbitraryAxis=[0 0 1]  RotationSequenceAxes=FollowerAxes  RotationSequence=XYX  RotationSequenceAngles=[0 0 0]  RotationSequenceAnglesUnits=rad  RotationMatrix=[1 0 0;0 1 0;0 0 1]  Quaternion=[1 0 0 0]  TranslationMethod=None  TranslationCartesianOffset=[0.03; -0.025; 0.0]  TranslationCartesianOffsetUnits=m  TranslationStandardAxis=+X  TranslationStandardOffset=0.035  TranslationStandardOffsetUnits=m  TranslationROffset=0  TranslationROffsetUnits=m  TranslationThetaOffset=0  TranslationThetaOffsetUnits=deg  TranslationZOffset=0  TranslationZOffsetUnits=m
  Simulink-PS Converter{1..5} (5 alike) : nesl_utility/Simulink-PS Converter  PhysicalDomain=network_engine_domain  SubClassName=ps_input  LeftPortType=input  RightPortType=output  PseudoPeriodic=off  Frequencies=[]  NoiseDistribution=none  NoiseParameters=[]  Unit=1  AffineConversion=off  FilteringAndDerivatives=filter  SimscapeFilterOrder=2  InputFilterTimeConstant=0.001  UdotUserProvided=0
  Spatial Contact Force : sm_lib/Forces and Torques/Spatial Contact Force  SenseSeparationDistance=off  NormalForceType=SmoothSpringDamper  NormalStiffness=cont_stiff  NormalStiffnessUnits=N/m  NormalDamping=cont_damp  NormalDampingUnits=N/(m/s)  NormalTransitionRegionWidth=cont_tranReg  NormalTransitionRegionWidthUnits=m  FrictionType=SmoothStickSlip  CoefficientOfStaticFriction=sf  CoefficientOfDynamicFriction=df  FrictionalCriticalVelocity=1e-3  FrictionalCriticalVelocityUnits=m/s  SenseContactSignal=off  SensePenetrationDepth=off  SenseNormalVelocity=off  SenseTangentialVelocity=off  SensingForceTorqueDirection=BaseOnFollower  SensingForceTorqueResolutionFrame=ContactFrame  SenseNormalForce=off  SenseNormalForceMagnitude=off  SenseNormalTorque=off  SenseFrictionalForce=off  SenseFrictionalForceMagnitude=off  SenseFrictionalTorque=off  SenseTotalForce=off  SenseTotalTorque=off  SenseContactBaseRotation=off  SenseContactBaseTranslation=off  SenseContactFollowerRotation=off  SenseContactFollowerTranslation=off  ZeroCrossDetectContactStartAndEnd=off
  Spatial Contact Force1 : sm_lib/Forces and Torques/Spatial Contact Force  SenseSeparationDistance=off  NormalForceType=SmoothSpringDamper  NormalStiffness=cont_stiff  NormalStiffnessUnits=N/m  NormalDamping=cont_damp  NormalDampingUnits=N/(m/s)  NormalTransitionRegionWidth=cont_tranReg  NormalTransitionRegionWidthUnits=m  FrictionType=SmoothStickSlip  CoefficientOfStaticFriction=sf  CoefficientOfDynamicFriction=df  FrictionalCriticalVelocity=1e-3  FrictionalCriticalVelocityUnits=m/s  SenseContactSignal=off  SensePenetrationDepth=off  SenseNormalVelocity=off  SenseTangentialVelocity=off  SensingForceTorqueDirection=BaseOnFollower  SensingForceTorqueResolutionFrame=ContactFrame  SenseNormalForce=off  SenseNormalForceMagnitude=off  SenseNormalTorque=off  SenseFrictionalForce=off  SenseFrictionalForceMagnitude=off  SenseFrictionalTorque=off  SenseTotalForce=off  SenseTotalTorque=off  SenseContactBaseRotation=off  SenseContactBaseTranslation=off  SenseContactFollowerRotation=off  SenseContactFollowerTranslation=off  ZeroCrossDetectContactStartAndEnd=off
  Spatial Contact Force2 : sm_lib/Forces and Torques/Spatial Contact Force  SenseSeparationDistance=off  NormalForceType=SmoothSpringDamper  NormalStiffness=cont_stiff  NormalStiffnessUnits=N/m  NormalDamping=cont_damp  NormalDampingUnits=N/(m/s)  NormalTransitionRegionWidth=cont_tranReg  NormalTransitionRegionWidthUnits=m  FrictionType=SmoothStickSlip  CoefficientOfStaticFriction=sf  CoefficientOfDynamicFriction=df  FrictionalCriticalVelocity=1e-3  FrictionalCriticalVelocityUnits=m/s  SenseContactSignal=off  SensePenetrationDepth=off  SenseNormalVelocity=off  SenseTangentialVelocity=off  SensingForceTorqueDirection=BaseOnFollower  SensingForceTorqueResolutionFrame=ContactFrame  SenseNormalForce=off  SenseNormalForceMagnitude=off  SenseNormalTorque=off  SenseFrictionalForce=off  SenseFrictionalForceMagnitude=off  SenseFrictionalTorque=off  SenseTotalForce=off  SenseTotalTorque=off  SenseContactBaseRotation=off  SenseContactBaseTranslation=off  SenseContactFollowerRotation=off  SenseContactFollowerTranslation=off  ZeroCrossDetectContactStartAndEnd=off
  Spatial Contact Force3 : sm_lib/Forces and Torques/Spatial Contact Force  SenseSeparationDistance=off  NormalForceType=SmoothSpringDamper  NormalStiffness=cont_stiff  NormalStiffnessUnits=N/m  NormalDamping=cont_damp  NormalDampingUnits=N/(m/s)  NormalTransitionRegionWidth=cont_tranReg  NormalTransitionRegionWidthUnits=m  FrictionType=SmoothStickSlip  CoefficientOfStaticFriction=sf  CoefficientOfDynamicFriction=df  FrictionalCriticalVelocity=1e-3  FrictionalCriticalVelocityUnits=m/s  SenseContactSignal=on  SensePenetrationDepth=off  SenseNormalVelocity=off  SenseTangentialVelocity=off  SensingForceTorqueDirection=BaseOnFollower  SensingForceTorqueResolutionFrame=ContactFrame  SenseNormalForce=off  SenseNormalForceMagnitude=off  SenseNormalTorque=off  SenseFrictionalForce=off  SenseFrictionalForceMagnitude=off  SenseFrictionalTorque=off  SenseTotalForce=off  SenseTotalTorque=off  SenseContactBaseRotation=off  SenseContactBaseTranslation=off  SenseContactFollowerRotation=off  SenseContactFollowerTranslation=off  ZeroCrossDetectContactStartAndEnd=off
  Subsystem3 : snake_single_module_library/Subsystem  SystemSampleTime=-1  VariantActivationTime=update diagram  EmptyChoice=off  PassThrough=off  PassThroughVariantControl=(default)  EmptyChoiceVariantControl=(default)  AllowFlexibleInterface=on  Latency=0  AutoFrameSizeCalculation=off
  back right : snake_single_module_library/Subsystem  SystemSampleTime=-1  VariantActivationTime=update diagram  EmptyChoice=off  PassThrough=off  PassThroughVariantControl=(default)  EmptyChoiceVariantControl=(default)  AllowFlexibleInterface=on  Latency=0  AutoFrameSizeCalculation=off
  base : PMIOPort  Side=Left
  contact : PMIOPort  Port=2  Side=Left
  isContact : Outport
  wires:
  theta_FL/1 -> Front Left/1
  theta_FR/1 -> Front right/1
  theta_BL/1 -> Back left/1
  theta_BR/1 -> back right/1
  theta_body/1 -> Subsystem3/1
  Gain1/1 -> Gain2/1
  Gain2/1 -> Simulink-PS Converter1/1
  phi_FL/1 -> Gain1/1
  Gain4/1 -> Simulink-PS Converter2/1
  Gain3/1 -> Gain4/1
  Gain5/1 -> Gain6/1
  Gain6/1 -> Simulink-PS Converter3/1
  Gain8/1 -> Simulink-PS Converter4/1
  Gain7/1 -> Gain8/1
  phi_FR/1 -> Gain3/1
  phi_BR/1 -> Gain7/1
  phi_BL/1 -> Gain5/1
  Gain10/1 -> Simulink-PS Converter5/1
  Gain9/1 -> Gain10/1
  phi_body/1 -> Gain9/1
  PS-Simulink Converter/1 -> isContact/1
  connections:
  Subsystem3/LConn3 -- contact/RConn1 -- Spatial Contact Force3/RConn1 -- back right/LConn3 -- Spatial Contact Force1/RConn1 -- Front right/LConn3 -- Spatial Contact Force2/RConn1 -- Back left/LConn3 -- Spatial Contact Force/RConn1 -- Front Left/LConn3
  Rigid Transform13/RConn1 -- File Solid3/RConn1
  back right/RConn1 -- Rigid Transform12/LConn1
  Rigid Transform5/RConn1 -- Rigid Transform8/LConn1
  Rigid Transform9/RConn1 -- Back left/LConn2
  Spatial Contact Force1/LConn1 -- File Solid1/LConn1
  Spatial Contact Force2/LConn1 -- File Solid3/LConn1
  Rigid Transform4/RConn1 -- Rigid Transform9/LConn1
  Subsystem3/RConn1 -- Rigid Transform4/LConn1 -- Rigid Transform5/LConn1
  Rigid Transform3/RConn1 -- Rigid Transform7/LConn1
  Front Left/LConn2 -- Rigid Transform6/RConn1
  Rigid Transform1/LConn1 -- base/RConn1 -- Rigid Transform3/LConn1 -- Subsystem3/LConn2
  Rigid Transform10/LConn1 -- Front Left/RConn1
  File Solid1/RConn1 -- Rigid Transform11/RConn1
  Rigid Transform8/RConn1 -- back right/LConn2
  Rigid Transform7/RConn1 -- Front right/LConn2
  Rigid Transform6/LConn1 -- Rigid Transform1/RConn1
  File Solid/RConn1 -- Spatial Contact Force/LConn1
  File Solid2/RConn1 -- Rigid Transform12/RConn1
  Rigid Transform10/RConn1 -- File Solid/LConn1
  Back left/RConn1 -- Rigid Transform13/LConn1
  Front right/RConn1 -- Rigid Transform11/LConn1
  Spatial Contact Force3/LConn1 -- File Solid2/LConn2
  Simulink-PS Converter1/RConn1 -- Front Left/LConn1
  Front right/LConn1 -- Simulink-PS Converter2/RConn1
  Back left/LConn1 -- Simulink-PS Converter3/RConn1
  back right/LConn1 -- Simulink-PS Converter4/RConn1
  Subsystem3/LConn1 -- Simulink-PS Converter5/RConn1
  Spatial Contact Force3/RConn2 -- PS-Simulink Converter/LConn1

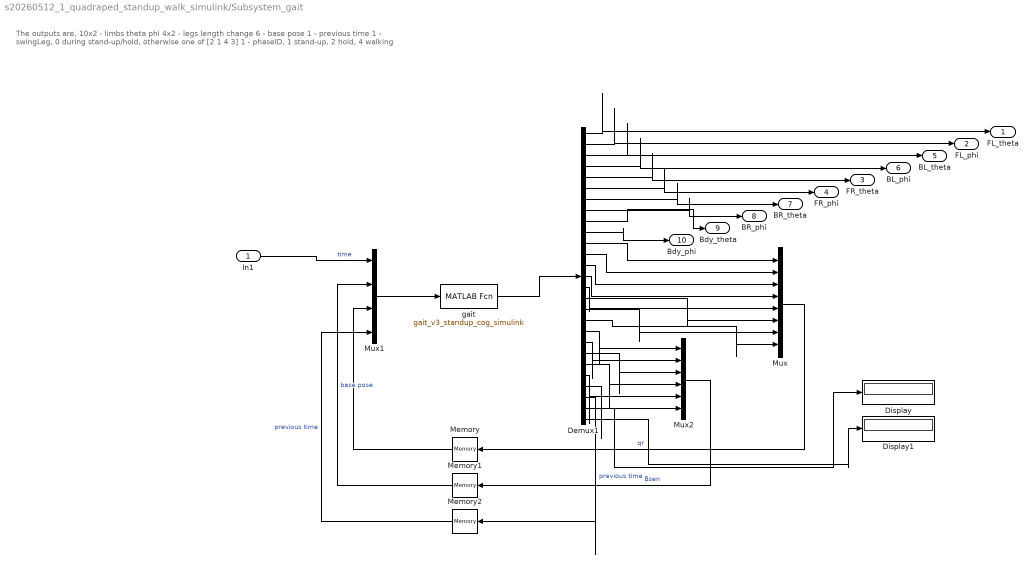
== system s20260512_1_quadraped_standup_walk_simulink/Subsystem_gait ==
  note: The outputs are,
      | 10x2 - limbs theta phi
      | 4x2 - legs length change
      | 6 - base pose
      | 1 - previous time
      | 1 - swingLeg, 0 during stand-up/hold, otherwise one of [2 1 4 3]
      | 1 - phaseID, 1 stand-up, 2 hold, 4 walking
  In1 : Inport
  Demux1 : Demux  Outputs=27
  Display : Display
  Display1 : Display
  Memory : Memory  InitialCondition=[0.0;0.0;0.0;0.0;0.0;0.0;0.0;0.0]
  Memory1 : Memory  InitialCondition=[0.0;0.0;0.0;0.0;0.0;0.0]
  Memory2 : Memory
  Mux : Mux  Inputs=8
  Mux1 : Mux
  Mux2 : Mux  Inputs=6
  gait : MATLABFcn  MATLABFcn=gait_v3_standup_cog_simulink  OutputDimensions=27
  FL_theta : Outport
  FL_phi : Outport  Port=2
  FR_theta : Outport  Port=3
  FR_phi : Outport  Port=4
  BL_theta : Outport  Port=5
  BL_phi : Outport  Port=6
  BR_theta : Outport  Port=7
  BR_phi : Outport  Port=8
  Bdy_theta : Outport  Port=9
  Bdy_phi : Outport  Port=10
  wires:
  Memory/1 -> Mux1/3
  Mux1/1 -> gait/1
  In1/1 -> Mux1/1  "time"
  gait/1 -> Demux1/1
  Mux/1 -> Memory/1  "qr"
  Demux1/1 -> FL_theta/1
  Demux1/2 -> FL_phi/1
  Demux1/3 -> BL_theta/1
  Demux1/4 -> BL_phi/1
  Demux1/5 -> FR_theta/1
  Demux1/6 -> FR_phi/1
  Demux1/7 -> BR_theta/1
  Demux1/8 -> BR_phi/1
  Mux2/1 -> Memory1/1  "Bsen"
  Memory1/1 -> Mux1/2  "base pose"
  Demux1/9 -> Bdy_theta/1
  Demux1/10 -> Bdy_phi/1
  Memory2/1 -> Mux1/4  "previous time"
  Demux1/11 -> Mux/1
  Demux1/12 -> Mux/2
  Demux1/13 -> Mux/3
  Demux1/14 -> Mux/4
  Demux1/15 -> Mux/5
  Demux1/16 -> Mux/6
  Demux1/17 -> Mux/7
  Demux1/18 -> Mux/8
  Demux1/19 -> Mux2/1
  Demux1/20 -> Mux2/2
  Demux1/21 -> Mux2/3
  Demux1/22 -> Mux2/4
  Demux1/23 -> Mux2/5
  Demux1/24 -> Mux2/6
  Demux1/25 -> Memory2/1  "previous time"
  Demux1/26 -> Display/1
  Demux1/27 -> Display1/1

== matlab function s20260512_1_quadraped_standup_walk_simulink/MATLAB Function ==
  data: t input; FL output; B input; qr input; contact input; BL output; FR output; BR output; qr output
function [FL, BL, FR, BR, qr] = gait(t, B, qr, contact)
%#codegen
persistent L r k T dt count legseq legs b straight_pose dp_cog isInitialized isTouched JC J npoints stepLen_l stepLen_r lift qr_initial

% robots parameters and the motion parameters
if isempty(L) && isempty(r) && isempty(k) && isempty(T) && isempty(dt) && isempty(isInitialized)
    L = 0.3175;   % length of the module
    r  = 0.013;   % radial offset of the 
    k = 9; % constraint legs
    T = 1; % swing time
    dt = 0.001; % descretization
    count =1; % iteration count
    legseq=[2,1,4,3]; % leg sequence
    legs = 2; % initial leg
    b = -2e-8*ones(2,1); % body bending
    straight_pose = 1e-8*ones(2,1); % length changes for straigt pose
    dp_cog = [0.0001;-0.00000;0.00000]; % CoG trajectory
    
    npoints = round(T/dt);
    tvec = 0:dt:T;

    stepLen_l = 0.04; % step length
    lift    = 0.01;
    gait_l = swingTrajectory_timeDependant(stepLen_l, lift, r, L, T, 0.0); % initial foot position
    
    
    stepLen_r = 0.04; % step length
    lift    = 0.01;
    gait_r = swingTrajectory_timeDependant(stepLen_r, lift, r, L, T, 0.0); % initial foot position

    H = gait_l(1,1); % the leg's X is worldframe Z. So the standing position.
    B(:,1) = [0;0;H; 0;0;0];  % [x y z roll pitch yaw] or your convention    
    
    % [l,~] = task2length([H; 0], r, L);
    % [l2,~] = task2length([gait_l(1,1); gait_l(2,1)], r, L);
    qr(:,1) = [0.009230935630945; 0.009230935630945; 0.007570474340197; 0.010946512434626; 0.009230935630945; 0.009230935630945; 0.009230935630945; 0.009230935630945];
    qr_initial = qr;
    
    isInitialized = true;
    isTouched = false;
    P_d_w = zeros(4,2);

    JC = zeros(k, 14);
    J = zeros(3, 14);
end

if contact == 1 && ~isTouched
    isTouched = true;
end

if isTouched

    if legs==1
        P_d_l = swingTrajectory_timeDependant(stepLen_l, lift, r, L, T, [t,t+dt] );
        Tbase = global_leg1HTM(straight_pose, 0.0, B, b, 0.0, L, r);
        P_d_w = Tbase * P_d_l;
        P_d_w = P_d_w(1:3,:);
    elseif legs ==2
        P_d_l = swingTrajectory_timeDependant(stepLen_l, lift, r, L, T, [t,t+dt] );
        Tbase = global_leg2HTM(straight_pose, 0.0, B, b, 1.0, L, r);
        P_d_w = Tbase * P_d_l;
        P_d_w = P_d_w(1:3,:);
    elseif legs==3
        flipy = eye(4);
        flipy(2,2) = -1;
        P_d_r = swingTrajectory_timeDependant(stepLen_r, lift, r, L, T, [t,t+dt] );
        Tbase = global_leg3HTM(straight_pose, 0.0, B, b, 0.0, L, r);
        P_d_w = Tbase * flipy * P_d_r;
        P_d_w = P_d_w(1:3,:);
    elseif legs==4
        flipy = eye(4);
        flipy(2,2) = -1;
        P_d_r = swingTrajectory_timeDependant(stepLen_r, lift, r, L, T, [t,t+dt] );
        Tbase = global_leg4HTM(straight_pose, 0.0, B, b, 1.0, L, r);
        P_d_w = Tbase * flipy * P_d_r;
        P_d_w = P_d_w(1:3,:);
    end
    
    jc1 = Jacobian_leg1(qr(1:2, 1), 1, B, b, 0.0, L, r);
    jc2 = Jacobian_leg2(qr(3:4, 1), 1, B, b, 1.0, L, r);
    jc3 = Jacobian_leg3(qr(5:6, 1), 1, B, b, 0.0, L, r);
    jc4 = Jacobian_leg4(qr(7:8, 1), 1, B, b, 1.0, L, r);
    
    % unconstraint leg
    if legs==1
        JC = [jc2; jc3; jc4];
        J = jc1;
    elseif legs ==2
        JC = [jc1; jc3; jc4];
        J = jc2;
    elseif legs==3
        JC = [jc1; jc2; jc4];
        J = jc3;
    elseif legs==4
        JC = [jc1; jc2; jc3];
        J = jc4;
    end

    Jcog = Jacobian_cog(qr(1:8), 1, B, b, 1.0, L, r);
    
    dp = P_d_w(:,2) - P_d_w(:,1);
    
    JJ = [JC;J;Jcog];
    W = diag([1000*ones(k, 1);100*ones(3,1); 10*ones(3,1)]);
    qr(:, 1) = qr(:, 1) + [eye(8), zeros(8,6)] * ( (W*JJ) \ (W * [zeros(k,1); dp; dp_cog]) );
    
    count =  count + 1;
    
    leg_idx = mod(floor((count-1)/npoints), numel(legseq)) + 1;
    legs = legseq(leg_idx);

    FL = length2config(qr(1:2, 1), r);
    BL = length2config(qr(3:4, 1), r);
    FR = length2config(qr(5:6, 1), r);
    BR = length2config(qr(7:8, 1), r);

else
    qr_initial = [0.009230935630945; 0.009230935630945; 0.007570474340197; 0.010946512434626; 0.009230935630945; 0.009230935630945; 0.009230935630945; 0.009230935630945];

    FL = length2config(qr_initial(1:2, 1), r);
    BL = length2config(qr_initial(3:4, 1), r);
    FR = length2config(qr_initial(5:6, 1), r);
    BR = length2config(qr_initial(7:8, 1), r);
    
end % end of the checking touch

end % end of the function
